simulink model "sim_estimator"  (R2024b)
settings: Solver=ode4  StartTime=t_0  StopTime=t_f  FixedStep=dt  RelTol=1e-8
settings Model: Creator=yevge  LastModifiedBy=yevge
settings DebuggingCC: AlgebraicLoopMsg=error  CheckMatrixSingularityMsg=error

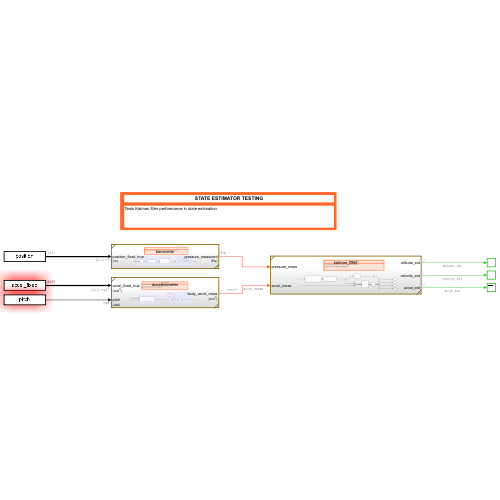
[thumbnail: Simulink's stored preview of the top-level diagram]
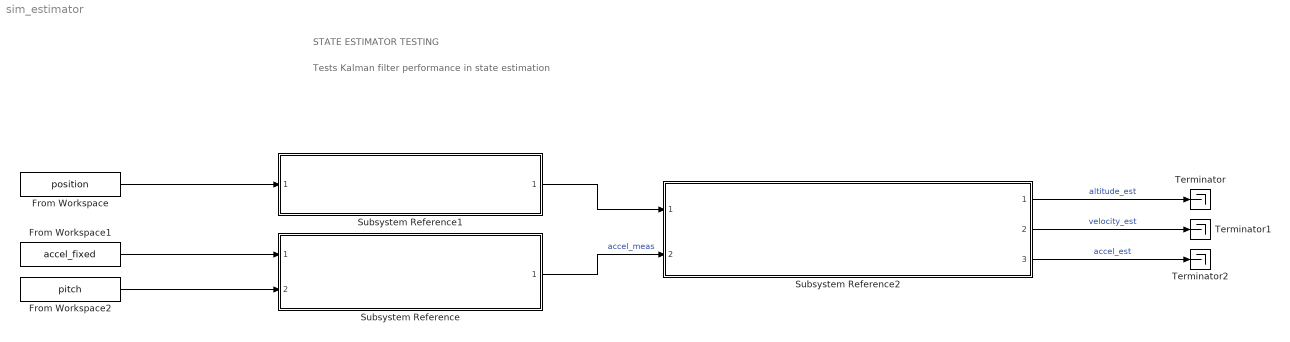
== system sim_estimator ==
  note: Tests Kalman filter performance in state estimation
  note: STATE ESTIMATOR TESTING
  From Workspace : FromWorkspace  VariableName=position
  From Workspace1 : FromWorkspace  VariableName=accel_fixed
  From Workspace2 : FromWorkspace  VariableName=pitch
  Subsystem Reference : Subsystem  ReferencedSubsystem=accelerometer
  Subsystem Reference1 : Subsystem  ReferencedSubsystem=barometer
  Subsystem Reference2 : Subsystem  ReferencedSubsystem=kalman_filter
  Terminator : Terminator
  Terminator1 : Terminator
  Terminator2 : Terminator
  wires:
  From Workspace/1 -> Subsystem Reference1/1
  From Workspace1/1 -> Subsystem Reference/1
  From Workspace2/1 -> Subsystem Reference/2
  Subsystem Reference/1 -> Subsystem Reference2/2  "accel_meas"
  Subsystem Reference1/1 -> Subsystem Reference2/1
  Subsystem Reference2/1 -> Terminator/1  "altitude_est"
  Subsystem Reference2/2 -> Terminator1/1  "velocity_est"
  Subsystem Reference2/3 -> Terminator2/1  "accel_est"
